simulink model "model_min_mine"  (R2018a)
settings: Solver=ode45  StartTime=0.0  StopTime=20  RelTol=1e-3
(part 9 of 10)

== system model_min_mine/5 систем підйому/6/7-періодні/7-ми періодна пр/Subsystem3 ==
  t1 : Inport
  t : Inport  Port=2
  a1 : Inport  Port=3
  Constant5 : Constant
  Scope2 : Scope
  Sum4 : Sum  Inputs=|+-  SaturateOnIntegerOverflow=on
  Switch1 : Switch  Criteria=u2 ~= 0  RndMeth=Zero  SaturateOnIntegerOverflow=on
  Генераці : Subsystem  TreatAsAtomicUnit=on
  Out1 : Outport
  wires:
  Генераці/1(Out1) -> Switch1/2
  Sum4/1 -> Генераці/Trigger
  Constant5/1 -> Генераці/1(In1)
  t/1 -> Sum4/2
  t1/1 -> Sum4/1
  Switch1/1 -> Out1/1, Scope2/1
  a1/1 -> Switch1/1

== system model_min_mine/5 систем підйому/6/7-періодні/7-ми періодна пр/Subsystem6 ==
  Сума t : Inport
  t : Inport  Port=2
  a : Inport  Port=3
  Constant5 : Constant
  Sum4 : Sum  Inputs=|+-  SaturateOnIntegerOverflow=on
  Switch1 : Switch  Criteria=u2 ~= 0  RndMeth=Zero  SaturateOnIntegerOverflow=on
  Генераці : Subsystem  TreatAsAtomicUnit=on
  Out1 : Outport
  wires:
  Генераці/1(Out1) -> Switch1/2
  Sum4/1 -> Генераці/Trigger
  Constant5/1 -> Генераці/1(In1)
  t/1 -> Sum4/2
  Сума t/1 -> Sum4/1
  Switch1/1 -> Out1/1
  a/1 -> Switch1/3

== system model_min_mine/5 систем підйому/6/7-періодні/7-ми періодна пр/Допоміжний ==
  t1 : Inport
  t : Inport  Port=2
  a1 : Inport  Port=3
  Constant5 : Constant
  Scope2 : Scope
  Sum4 : Sum  Inputs=|+-  SaturateOnIntegerOverflow=on
  Switch1 : Switch  Criteria=u2 ~= 0  RndMeth=Zero  SaturateOnIntegerOverflow=on
  Генераці : Subsystem  TreatAsAtomicUnit=on
  Out1 : Outport
  wires:
  Генераці/1(Out1) -> Switch1/2
  Sum4/1 -> Генераці/Trigger
  Constant5/1 -> Генераці/1(In1)
  t/1 -> Sum4/2
  t1/1 -> Sum4/1
  Switch1/1 -> Out1/1, Scope2/1
  a1/1 -> Switch1/1

== system model_min_mine/5 систем підйому/6/7-періодні/7-ми періодна пр/Допоміжний1 ==
  t1 : Inport
  t : Inport  Port=2
  a1 : Inport  Port=3
  Constant5 : Constant
  Scope2 : Scope
  Sum4 : Sum  Inputs=|+-  SaturateOnIntegerOverflow=on
  Switch1 : Switch  Criteria=u2 ~= 0  RndMeth=Zero  SaturateOnIntegerOverflow=on
  Генераці : Subsystem  TreatAsAtomicUnit=on
  Out1 : Outport
  wires:
  Генераці/1(Out1) -> Switch1/2
  Sum4/1 -> Генераці/Trigger
  Constant5/1 -> Генераці/1(In1)
  t/1 -> Sum4/2
  t1/1 -> Sum4/1
  Switch1/1 -> Out1/1, Scope2/1
  a1/1 -> Switch1/3

== system model_min_mine/5 систем підйому/6/7-періодні/7-ми періодна пр/постійні ==
  Sum1 : Sum  Inputs=|+++++++  SaturateOnIntegerOverflow=on
  Sum2 : Sum  Inputs=|+++  SaturateOnIntegerOverflow=on
  Sum3 : Sum  Inputs=|+++  SaturateOnIntegerOverflow=on
  Sum4 : Sum  Inputs=|++  SaturateOnIntegerOverflow=on
  a1 : Constant  Value=0.5
  a2 : Constant  Value=1.5
  "a4 " : Constant  Value=-1.5
  a5 : Constant  Value=-0.5
  t1 : Constant  Value=0.5
  "t1/ " : Constant  Value=0.5
  t2 : Constant  Value=3.5
  t3 : Constant  Value=8
  t4 : Constant  Value=3.5
  "t4/ " : Constant  Value=0.5
  t5 : Constant  Value=0.5
  Out1 : Outport
  Out2 : Outport  Port=2
  Out3 : Outport  Port=3
  Out4 : Outport  Port=4
  Out5 : Outport  Port=5
  Out6 : Outport  Port=6
  Out7 : Outport  Port=7
  Out8 : Outport  Port=8
  Out9 : Outport  Port=9
  Out10 : Outport  Port=10
  Out11 : Outport  Port=11
  wires:
  a1/1 -> Out1/1
  "a4 "/1 -> Out3/1
  a5/1 -> Out4/1
  a2/1 -> Out2/1
  t1/1 -> Out5/1, Sum1/1, Sum2/1, Sum4/1
  t3/1 -> Sum1/3, Sum2/3
  t2/1 -> Out6/1, Sum1/2, Sum2/2
  t5/1 -> Sum1/5
  t4/1 -> Out7/1, Sum1/4, Sum3/1
  Sum1/1 -> Out9/1
  Sum2/1 -> Out10/1, Sum3/2
  Sum3/1 -> Out8/1
  "t4/ "/1 -> Sum3/3, Sum1/6
  "t1/ "/1 -> Sum1/7, Sum4/2
  Sum4/1 -> Out11/1

== system model_min_mine/5 систем підйому/1/5-періодні/криво/Subsystem/Генераці ==
  In1 : Inport
  Trigger : TriggerPort  TriggerType=either  VariantControl=(inherit)  ShowOutputPort=on
  Out1 : Outport
  wires:
  In1/1 -> Out1/1

== system model_min_mine/5 систем підйому/1/5-періодні/криво/Subsystem1/Генераці ==
  In1 : Inport
  Trigger : TriggerPort  TriggerType=either  VariantControl=(inherit)  ShowOutputPort=on
  Out1 : Outport
  wires:
  In1/1 -> Out1/1

== system model_min_mine/5 систем підйому/1/5-періодні/криво/Subsystem2/Генераці ==
  In1 : Inport
  Trigger : TriggerPort  TriggerType=either  VariantControl=(inherit)  ShowOutputPort=on
  Out1 : Outport
  wires:
  In1/1 -> Out1/1

== system model_min_mine/5 систем підйому/1/5-періодні/криво/Subsystem3/Генераці ==
  In1 : Inport
  Trigger : TriggerPort  TriggerType=either  VariantControl=(inherit)  ShowOutputPort=on
  Out1 : Outport
  wires:
  In1/1 -> Out1/1

== system model_min_mine/5 систем підйому/1/5-періодні/криво/Subsystem6/Генераці ==
  In1 : Inport
  Trigger : TriggerPort  TriggerType=either  VariantControl=(inherit)  ShowOutputPort=on
  Out1 : Outport
  wires:
  In1/1 -> Out1/1

== system model_min_mine/5 систем підйому/1/5-періодні/криво/Допоміжний/Генераці ==
  In1 : Inport
  Trigger : TriggerPort  TriggerType=either  VariantControl=(inherit)  ShowOutputPort=on
  Out1 : Outport
  wires:
  In1/1 -> Out1/1

== system model_min_mine/5 систем підйому/1/5-періодні/криво/Допоміжний1/Генераці ==
  In1 : Inport
  Trigger : TriggerPort  TriggerType=either  VariantControl=(inherit)  ShowOutputPort=on
  Out1 : Outport
  wires:
  In1/1 -> Out1/1

== system model_min_mine/5 систем підйому/1/5-періодні/пр/Subsystem/Генераці ==
  In1 : Inport
  Trigger : TriggerPort  TriggerType=either  VariantControl=(inherit)  ShowOutputPort=on
  Out1 : Outport
  wires:
  In1/1 -> Out1/1

== system model_min_mine/5 систем підйому/1/5-періодні/пр/Subsystem1/Генераці ==
  In1 : Inport
  Trigger : TriggerPort  TriggerType=either  VariantControl=(inherit)  ShowOutputPort=on
  Out1 : Outport
  wires:
  In1/1 -> Out1/1

== system model_min_mine/5 систем підйому/1/5-періодні/пр/Subsystem4/Генераці ==
  In1 : Inport
  Trigger : TriggerPort  TriggerType=either  VariantControl=(inherit)  ShowOutputPort=on
  Out1 : Outport
  wires:
  In1/1 -> Out1/1

== system model_min_mine/5 систем підйому/1/5-періодні/пр/Subsystem5/Генераці ==
  In1 : Inport
  Trigger : TriggerPort  TriggerType=either  VariantControl=(inherit)  ShowOutputPort=on
  Out1 : Outport
  wires:
  In1/1 -> Out1/1

== system model_min_mine/5 систем підйому/1/5-періодні/пр/Subsystem6/Генераці ==
  In1 : Inport
  Trigger : TriggerPort  TriggerType=either  VariantControl=(inherit)  ShowOutputPort=on
  Out1 : Outport
  wires:
  In1/1 -> Out1/1

== system model_min_mine/5 систем підйому/1/5-періодні/пр/Допоміжний/Генераці ==
  In1 : Inport
  Trigger : TriggerPort  TriggerType=either  VariantControl=(inherit)  ShowOutputPort=on
  Out1 : Outport
  wires:
  In1/1 -> Out1/1

== system model_min_mine/5 систем підйому/1/5-періодні/пр/Допоміжний -1/Генераці ==
  In1 : Inport
  Trigger : TriggerPort  TriggerType=either  VariantControl=(inherit)  ShowOutputPort=on
  Out1 : Outport
  wires:
  In1/1 -> Out1/1

== system model_min_mine/5 систем підйому/1/5-періодні/пр/Допоміжний -2/Генераці ==
  In1 : Inport
  Trigger : TriggerPort  TriggerType=either  VariantControl=(inherit)  ShowOutputPort=on
  Out1 : Outport
  wires:
  In1/1 -> Out1/1

== system model_min_mine/5 систем підйому/1/5-періодні/пр/Допоміжний -3/Генераці ==
  In1 : Inport
  Trigger : TriggerPort  TriggerType=either  VariantControl=(inherit)  ShowOutputPort=on
  Out1 : Outport
  wires:
  In1/1 -> Out1/1

== system model_min_mine/5 систем підйому/1/5-періодні/пр/Допоміжний -4/Генераці ==
  In1 : Inport
  Trigger : TriggerPort  TriggerType=either  VariantControl=(inherit)  ShowOutputPort=on
  Out1 : Outport
  wires:
  In1/1 -> Out1/1

== system model_min_mine/5 систем підйому/1/6-періодні/6-ти періодна криволінійна/Subsystem/Генераці ==
  In1 : Inport
  Trigger : TriggerPort  TriggerType=either  VariantControl=(inherit)  ShowOutputPort=on
  Out1 : Outport
  wires:
  In1/1 -> Out1/1

== system model_min_mine/5 систем підйому/1/6-періодні/6-ти періодна криволінійна/Subsystem3/Генераці ==
  In1 : Inport
  Trigger : TriggerPort  TriggerType=either  VariantControl=(inherit)  ShowOutputPort=on
  Out1 : Outport
  wires:
  In1/1 -> Out1/1

== system model_min_mine/5 систем підйому/1/6-періодні/6-ти періодна криволінійна/Subsystem6/Генераці ==
  In1 : Inport
  Trigger : TriggerPort  TriggerType=either  VariantControl=(inherit)  ShowOutputPort=on
  Out1 : Outport
  wires:
  In1/1 -> Out1/1

== system model_min_mine/5 систем підйому/1/6-періодні/6-ти періодна криволінійна/Допоміжний/Генераці ==
  In1 : Inport
  Trigger : TriggerPort  TriggerType=either  VariantControl=(inherit)  ShowOutputPort=on
  Out1 : Outport
  wires:
  In1/1 -> Out1/1

== system model_min_mine/5 систем підйому/1/6-періодні/6-ти періодна криволінійна/Допоміжний1/Генераці ==
  In1 : Inport
  Trigger : TriggerPort  TriggerType=either  VariantControl=(inherit)  ShowOutputPort=on
  Out1 : Outport
  wires:
  In1/1 -> Out1/1

== system model_min_mine/5 систем підйому/1/6-періодні/6-ти періодна пр/Subsystem/Генераці ==
  In1 : Inport
  Trigger : TriggerPort  TriggerType=either  VariantControl=(inherit)  ShowOutputPort=on
  Out1 : Outport
  wires:
  In1/1 -> Out1/1

== system model_min_mine/5 систем підйому/1/6-періодні/6-ти періодна пр/Subsystem1/Генераці ==
  In1 : Inport
  Trigger : TriggerPort  TriggerType=either  VariantControl=(inherit)  ShowOutputPort=on
  Out1 : Outport
  wires:
  In1/1 -> Out1/1

== system model_min_mine/5 систем підйому/1/6-періодні/6-ти періодна пр/Subsystem2/Генераці ==
  In1 : Inport
  Trigger : TriggerPort  TriggerType=either  VariantControl=(inherit)  ShowOutputPort=on
  Out1 : Outport
  wires:
  In1/1 -> Out1/1

== system model_min_mine/5 систем підйому/1/6-періодні/6-ти періодна пр/Subsystem3/Генераці ==
  In1 : Inport
  Trigger : TriggerPort  TriggerType=either  VariantControl=(inherit)  ShowOutputPort=on
  Out1 : Outport
  wires:
  In1/1 -> Out1/1

== system model_min_mine/5 систем підйому/1/6-періодні/6-ти періодна пр/Subsystem6/Генераці ==
  In1 : Inport
  Trigger : TriggerPort  TriggerType=either  VariantControl=(inherit)  ShowOutputPort=on
  Out1 : Outport
  wires:
  In1/1 -> Out1/1

== system model_min_mine/5 систем підйому/1/6-періодні/6-ти періодна пр/Допоміжний/Генераці ==
  In1 : Inport
  Trigger : TriggerPort  TriggerType=either  VariantControl=(inherit)  ShowOutputPort=on
  Out1 : Outport
  wires:
  In1/1 -> Out1/1

== system model_min_mine/5 систем підйому/1/6-періодні/6-ти періодна пр/Допоміжний1/Генераці ==
  In1 : Inport
  Trigger : TriggerPort  TriggerType=either  VariantControl=(inherit)  ShowOutputPort=on
  Out1 : Outport
  wires:
  In1/1 -> Out1/1

== system model_min_mine/5 систем підйому/1/7-періодні/7-ми періодна криволінійна/Subsystem/Генераці ==
  In1 : Inport
  Trigger : TriggerPort  TriggerType=either  VariantControl=(inherit)  ShowOutputPort=on
  Out1 : Outport
  wires:
  In1/1 -> Out1/1

== system model_min_mine/5 систем підйому/1/7-періодні/7-ми періодна криволінійна/Subsystem3/Генераці ==
  In1 : Inport
  Trigger : TriggerPort  TriggerType=either  VariantControl=(inherit)  ShowOutputPort=on
  Out1 : Outport
  wires:
  In1/1 -> Out1/1

== system model_min_mine/5 систем підйому/1/7-періодні/7-ми періодна криволінійна/Subsystem6/Генераці ==
  In1 : Inport
  Trigger : TriggerPort  TriggerType=either  VariantControl=(inherit)  ShowOutputPort=on
  Out1 : Outport
  wires:
  In1/1 -> Out1/1

== system model_min_mine/5 систем підйому/1/7-періодні/7-ми періодна криволінійна/Допоміжний/Генераці ==
  In1 : Inport
  Trigger : TriggerPort  TriggerType=either  VariantControl=(inherit)  ShowOutputPort=on
  Out1 : Outport
  wires:
  In1/1 -> Out1/1

== system model_min_mine/5 систем підйому/1/7-періодні/7-ми періодна криволінійна/Допоміжний1/Генераці ==
  In1 : Inport
  Trigger : TriggerPort  TriggerType=either  VariantControl=(inherit)  ShowOutputPort=on
  Out1 : Outport
  wires:
  In1/1 -> Out1/1

== system model_min_mine/5 систем підйому/1/7-періодні/7-ми періодна пр/Subsystem/Генераці ==
  In1 : Inport
  Trigger : TriggerPort  TriggerType=either  VariantControl=(inherit)  ShowOutputPort=on
  Out1 : Outport
  wires:
  In1/1 -> Out1/1

== system model_min_mine/5 систем підйому/1/7-періодні/7-ми періодна пр/Subsystem1/Генераці ==
  In1 : Inport
  Trigger : TriggerPort  TriggerType=either  VariantControl=(inherit)  ShowOutputPort=on
  Out1 : Outport
  wires:
  In1/1 -> Out1/1

== system model_min_mine/5 систем підйому/1/7-періодні/7-ми періодна пр/Subsystem2/Генераці ==
  In1 : Inport
  Trigger : TriggerPort  TriggerType=either  VariantControl=(inherit)  ShowOutputPort=on
  Out1 : Outport
  wires:
  In1/1 -> Out1/1

== system model_min_mine/5 систем підйому/1/7-періодні/7-ми періодна пр/Subsystem3/Генераці ==
  In1 : Inport
  Trigger : TriggerPort  TriggerType=either  VariantControl=(inherit)  ShowOutputPort=on
  Out1 : Outport
  wires:
  In1/1 -> Out1/1

== system model_min_mine/5 систем підйому/1/7-періодні/7-ми періодна пр/Subsystem6/Генераці ==
  In1 : Inport
  Trigger : TriggerPort  TriggerType=either  VariantControl=(inherit)  ShowOutputPort=on
  Out1 : Outport
  wires:
  In1/1 -> Out1/1

== system model_min_mine/5 систем підйому/1/7-періодні/7-ми періодна пр/Допоміжний/Генераці ==
  In1 : Inport
  Trigger : TriggerPort  TriggerType=either  VariantControl=(inherit)  ShowOutputPort=on
  Out1 : Outport
  wires:
  In1/1 -> Out1/1

== system model_min_mine/5 систем підйому/1/7-періодні/7-ми періодна пр/Допоміжний1/Генераці ==
  In1 : Inport
  Trigger : TriggerPort  TriggerType=either  VariantControl=(inherit)  ShowOutputPort=on
  Out1 : Outport
  wires:
  In1/1 -> Out1/1

== system model_min_mine/5 систем підйому/2/5-періодні/криво/Subsystem/Генераці ==
  In1 : Inport
  Trigger : TriggerPort  TriggerType=either  VariantControl=(inherit)  ShowOutputPort=on
  Out1 : Outport
  wires:
  In1/1 -> Out1/1

== system model_min_mine/5 систем підйому/2/5-періодні/криво/Subsystem1/Генераці ==
  In1 : Inport
  Trigger : TriggerPort  TriggerType=either  VariantControl=(inherit)  ShowOutputPort=on
  Out1 : Outport
  wires:
  In1/1 -> Out1/1

== system model_min_mine/5 систем підйому/2/5-періодні/криво/Subsystem2/Генераці ==
  In1 : Inport
  Trigger : TriggerPort  TriggerType=either  VariantControl=(inherit)  ShowOutputPort=on
  Out1 : Outport
  wires:
  In1/1 -> Out1/1

== system model_min_mine/5 систем підйому/2/5-періодні/криво/Subsystem3/Генераці ==
  In1 : Inport
  Trigger : TriggerPort  TriggerType=either  VariantControl=(inherit)  ShowOutputPort=on
  Out1 : Outport
  wires:
  In1/1 -> Out1/1

== system model_min_mine/5 систем підйому/2/5-періодні/криво/Subsystem6/Генераці ==
  In1 : Inport
  Trigger : TriggerPort  TriggerType=either  VariantControl=(inherit)  ShowOutputPort=on
  Out1 : Outport
  wires:
  In1/1 -> Out1/1

== system model_min_mine/5 систем підйому/2/5-періодні/криво/Допоміжний/Генераці ==
  In1 : Inport
  Trigger : TriggerPort  TriggerType=either  VariantControl=(inherit)  ShowOutputPort=on
  Out1 : Outport
  wires:
  In1/1 -> Out1/1

== system model_min_mine/5 систем підйому/2/5-періодні/криво/Допоміжний1/Генераці ==
  In1 : Inport
  Trigger : TriggerPort  TriggerType=either  VariantControl=(inherit)  ShowOutputPort=on
  Out1 : Outport
  wires:
  In1/1 -> Out1/1

== system model_min_mine/5 систем підйому/2/5-періодні/пр/Subsystem/Генераці ==
  In1 : Inport
  Trigger : TriggerPort  TriggerType=either  VariantControl=(inherit)  ShowOutputPort=on
  Out1 : Outport
  wires:
  In1/1 -> Out1/1

== system model_min_mine/5 систем підйому/2/5-періодні/пр/Subsystem1/Генераці ==
  In1 : Inport
  Trigger : TriggerPort  TriggerType=either  VariantControl=(inherit)  ShowOutputPort=on
  Out1 : Outport
  wires:
  In1/1 -> Out1/1

== system model_min_mine/5 систем підйому/2/5-періодні/пр/Subsystem4/Генераці ==
  In1 : Inport
  Trigger : TriggerPort  TriggerType=either  VariantControl=(inherit)  ShowOutputPort=on
  Out1 : Outport
  wires:
  In1/1 -> Out1/1

== system model_min_mine/5 систем підйому/2/5-періодні/пр/Subsystem5/Генераці ==
  In1 : Inport
  Trigger : TriggerPort  TriggerType=either  VariantControl=(inherit)  ShowOutputPort=on
  Out1 : Outport
  wires:
  In1/1 -> Out1/1

== system model_min_mine/5 систем підйому/2/5-періодні/пр/Subsystem6/Генераці ==
  In1 : Inport
  Trigger : TriggerPort  TriggerType=either  VariantControl=(inherit)  ShowOutputPort=on
  Out1 : Outport
  wires:
  In1/1 -> Out1/1

== system model_min_mine/5 систем підйому/2/5-періодні/пр/Допоміжний/Генераці ==
  In1 : Inport
  Trigger : TriggerPort  TriggerType=either  VariantControl=(inherit)  ShowOutputPort=on
  Out1 : Outport
  wires:
  In1/1 -> Out1/1

== system model_min_mine/5 систем підйому/2/5-періодні/пр/Допоміжний -1/Генераці ==
  In1 : Inport
  Trigger : TriggerPort  TriggerType=either  VariantControl=(inherit)  ShowOutputPort=on
  Out1 : Outport
  wires:
  In1/1 -> Out1/1

== system model_min_mine/5 систем підйому/2/5-періодні/пр/Допоміжний -2/Генераці ==
  In1 : Inport
  Trigger : TriggerPort  TriggerType=either  VariantControl=(inherit)  ShowOutputPort=on
  Out1 : Outport
  wires:
  In1/1 -> Out1/1

== system model_min_mine/5 систем підйому/2/5-періодні/пр/Допоміжний -3/Генераці ==
  In1 : Inport
  Trigger : TriggerPort  TriggerType=either  VariantControl=(inherit)  ShowOutputPort=on
  Out1 : Outport
  wires:
  In1/1 -> Out1/1

== system model_min_mine/5 систем підйому/2/5-періодні/пр/Допоміжний -4/Генераці ==
  In1 : Inport
  Trigger : TriggerPort  TriggerType=either  VariantControl=(inherit)  ShowOutputPort=on
  Out1 : Outport
  wires:
  In1/1 -> Out1/1

== system model_min_mine/5 систем підйому/2/6-періодні/6-ти періодна криволінійна/Subsystem/Генераці ==
  In1 : Inport
  Trigger : TriggerPort  TriggerType=either  VariantControl=(inherit)  ShowOutputPort=on
  Out1 : Outport
  wires:
  In1/1 -> Out1/1

== system model_min_mine/5 систем підйому/2/6-періодні/6-ти періодна криволінійна/Subsystem3/Генераці ==
  In1 : Inport
  Trigger : TriggerPort  TriggerType=either  VariantControl=(inherit)  ShowOutputPort=on
  Out1 : Outport
  wires:
  In1/1 -> Out1/1

== system model_min_mine/5 систем підйому/2/6-періодні/6-ти періодна криволінійна/Subsystem6/Генераці ==
  In1 : Inport
  Trigger : TriggerPort  TriggerType=either  VariantControl=(inherit)  ShowOutputPort=on
  Out1 : Outport
  wires:
  In1/1 -> Out1/1

== system model_min_mine/5 систем підйому/2/6-періодні/6-ти періодна криволінійна/Допоміжний/Генераці ==
  In1 : Inport
  Trigger : TriggerPort  TriggerType=either  VariantControl=(inherit)  ShowOutputPort=on
  Out1 : Outport
  wires:
  In1/1 -> Out1/1

== system model_min_mine/5 систем підйому/2/6-періодні/6-ти періодна криволінійна/Допоміжний1/Генераці ==
  In1 : Inport
  Trigger : TriggerPort  TriggerType=either  VariantControl=(inherit)  ShowOutputPort=on
  Out1 : Outport
  wires:
  In1/1 -> Out1/1

== system model_min_mine/5 систем підйому/2/6-періодні/6-ти періодна пр/Subsystem/Генераці ==
  In1 : Inport
  Trigger : TriggerPort  TriggerType=either  VariantControl=(inherit)  ShowOutputPort=on
  Out1 : Outport
  wires:
  In1/1 -> Out1/1

== system model_min_mine/5 систем підйому/2/6-періодні/6-ти періодна пр/Subsystem1/Генераці ==
  In1 : Inport
  Trigger : TriggerPort  TriggerType=either  VariantControl=(inherit)  ShowOutputPort=on
  Out1 : Outport
  wires:
  In1/1 -> Out1/1

== system model_min_mine/5 систем підйому/2/6-періодні/6-ти періодна пр/Subsystem2/Генераці ==
  In1 : Inport
  Trigger : TriggerPort  TriggerType=either  VariantControl=(inherit)  ShowOutputPort=on
  Out1 : Outport
  wires:
  In1/1 -> Out1/1

== system model_min_mine/5 систем підйому/2/6-періодні/6-ти періодна пр/Subsystem3/Генераці ==
  In1 : Inport
  Trigger : TriggerPort  TriggerType=either  VariantControl=(inherit)  ShowOutputPort=on
  Out1 : Outport
  wires:
  In1/1 -> Out1/1

== system model_min_mine/5 систем підйому/2/6-періодні/6-ти періодна пр/Subsystem6/Генераці ==
  In1 : Inport
  Trigger : TriggerPort  TriggerType=either  VariantControl=(inherit)  ShowOutputPort=on
  Out1 : Outport
  wires:
  In1/1 -> Out1/1

== system model_min_mine/5 систем підйому/2/6-періодні/6-ти періодна пр/Допоміжний/Генераці ==
  In1 : Inport
  Trigger : TriggerPort  TriggerType=either  VariantControl=(inherit)  ShowOutputPort=on
  Out1 : Outport
  wires:
  In1/1 -> Out1/1

== system model_min_mine/5 систем підйому/2/6-періодні/6-ти періодна пр/Допоміжний1/Генераці ==
  In1 : Inport
  Trigger : TriggerPort  TriggerType=either  VariantControl=(inherit)  ShowOutputPort=on
  Out1 : Outport
  wires:
  In1/1 -> Out1/1

== system model_min_mine/5 систем підйому/2/7-періодні/7-ми періодна криволінійна/Subsystem/Генераці ==
  In1 : Inport
  Trigger : TriggerPort  TriggerType=either  VariantControl=(inherit)  ShowOutputPort=on
  Out1 : Outport
  wires:
  In1/1 -> Out1/1

== system model_min_mine/5 систем підйому/2/7-періодні/7-ми періодна криволінійна/Subsystem3/Генераці ==
  In1 : Inport
  Trigger : TriggerPort  TriggerType=either  VariantControl=(inherit)  ShowOutputPort=on
  Out1 : Outport
  wires:
  In1/1 -> Out1/1

== system model_min_mine/5 систем підйому/2/7-періодні/7-ми періодна криволінійна/Subsystem6/Генераці ==
  In1 : Inport
  Trigger : TriggerPort  TriggerType=either  VariantControl=(inherit)  ShowOutputPort=on
  Out1 : Outport
  wires:
  In1/1 -> Out1/1

== system model_min_mine/5 систем підйому/2/7-періодні/7-ми періодна криволінійна/Допоміжний/Генераці ==
  In1 : Inport
  Trigger : TriggerPort  TriggerType=either  VariantControl=(inherit)  ShowOutputPort=on
  Out1 : Outport
  wires:
  In1/1 -> Out1/1

== system model_min_mine/5 систем підйому/2/7-періодні/7-ми періодна криволінійна/Допоміжний1/Генераці ==
  In1 : Inport
  Trigger : TriggerPort  TriggerType=either  VariantControl=(inherit)  ShowOutputPort=on
  Out1 : Outport
  wires:
  In1/1 -> Out1/1

== system model_min_mine/5 систем підйому/2/7-періодні/7-ми періодна пр/Subsystem/Генераці ==
  In1 : Inport
  Trigger : TriggerPort  TriggerType=either  VariantControl=(inherit)  ShowOutputPort=on
  Out1 : Outport
  wires:
  In1/1 -> Out1/1

== system model_min_mine/5 систем підйому/2/7-періодні/7-ми періодна пр/Subsystem1/Генераці ==
  In1 : Inport
  Trigger : TriggerPort  TriggerType=either  VariantControl=(inherit)  ShowOutputPort=on
  Out1 : Outport
  wires:
  In1/1 -> Out1/1

== system model_min_mine/5 систем підйому/2/7-періодні/7-ми періодна пр/Subsystem2/Генераці ==
  In1 : Inport
  Trigger : TriggerPort  TriggerType=either  VariantControl=(inherit)  ShowOutputPort=on
  Out1 : Outport
  wires:
  In1/1 -> Out1/1

== system model_min_mine/5 систем підйому/2/7-періодні/7-ми періодна пр/Subsystem3/Генераці ==
  In1 : Inport
  Trigger : TriggerPort  TriggerType=either  VariantControl=(inherit)  ShowOutputPort=on
  Out1 : Outport
  wires:
  In1/1 -> Out1/1

== system model_min_mine/5 систем підйому/2/7-періодні/7-ми періодна пр/Subsystem6/Генераці ==
  In1 : Inport
  Trigger : TriggerPort  TriggerType=either  VariantControl=(inherit)  ShowOutputPort=on
  Out1 : Outport
  wires:
  In1/1 -> Out1/1

== system model_min_mine/5 систем підйому/2/7-періодні/7-ми періодна пр/Допоміжний/Генераці ==
  In1 : Inport
  Trigger : TriggerPort  TriggerType=either  VariantControl=(inherit)  ShowOutputPort=on
  Out1 : Outport
  wires:
  In1/1 -> Out1/1

== system model_min_mine/5 систем підйому/2/7-періодні/7-ми періодна пр/Допоміжний1/Генераці ==
  In1 : Inport
  Trigger : TriggerPort  TriggerType=either  VariantControl=(inherit)  ShowOutputPort=on
  Out1 : Outport
  wires:
  In1/1 -> Out1/1

== system model_min_mine/5 систем підйому/3/5-періодні/криво/Subsystem/Генераці ==
  In1 : Inport
  Trigger : TriggerPort  TriggerType=either  VariantControl=(inherit)  ShowOutputPort=on
  Out1 : Outport
  wires:
  In1/1 -> Out1/1

== system model_min_mine/5 систем підйому/3/5-періодні/криво/Subsystem1/Генераці ==
  In1 : Inport
  Trigger : TriggerPort  TriggerType=either  VariantControl=(inherit)  ShowOutputPort=on
  Out1 : Outport
  wires:
  In1/1 -> Out1/1

== system model_min_mine/5 систем підйому/3/5-періодні/криво/Subsystem2/Генераці ==
  In1 : Inport
  Trigger : TriggerPort  TriggerType=either  VariantControl=(inherit)  ShowOutputPort=on
  Out1 : Outport
  wires:
  In1/1 -> Out1/1

== system model_min_mine/5 систем підйому/3/5-періодні/криво/Subsystem3/Генераці ==
  In1 : Inport
  Trigger : TriggerPort  TriggerType=either  VariantControl=(inherit)  ShowOutputPort=on
  Out1 : Outport
  wires:
  In1/1 -> Out1/1

== system model_min_mine/5 систем підйому/3/5-періодні/криво/Subsystem6/Генераці ==
  In1 : Inport
  Trigger : TriggerPort  TriggerType=either  VariantControl=(inherit)  ShowOutputPort=on
  Out1 : Outport
  wires:
  In1/1 -> Out1/1

== system model_min_mine/5 систем підйому/3/5-періодні/криво/Допоміжний/Генераці ==
  In1 : Inport
  Trigger : TriggerPort  TriggerType=either  VariantControl=(inherit)  ShowOutputPort=on
  Out1 : Outport
  wires:
  In1/1 -> Out1/1

== system model_min_mine/5 систем підйому/3/5-періодні/криво/Допоміжний1/Генераці ==
  In1 : Inport
  Trigger : TriggerPort  TriggerType=either  VariantControl=(inherit)  ShowOutputPort=on
  Out1 : Outport
  wires:
  In1/1 -> Out1/1

== system model_min_mine/5 систем підйому/3/5-періодні/пр/Subsystem/Генераці ==
  In1 : Inport
  Trigger : TriggerPort  TriggerType=either  VariantControl=(inherit)  ShowOutputPort=on
  Out1 : Outport
  wires:
  In1/1 -> Out1/1

== system model_min_mine/5 систем підйому/3/5-періодні/пр/Subsystem1/Генераці ==
  In1 : Inport
  Trigger : TriggerPort  TriggerType=either  VariantControl=(inherit)  ShowOutputPort=on
  Out1 : Outport
  wires:
  In1/1 -> Out1/1

== system model_min_mine/5 систем підйому/3/5-періодні/пр/Subsystem4/Генераці ==
  In1 : Inport
  Trigger : TriggerPort  TriggerType=either  VariantControl=(inherit)  ShowOutputPort=on
  Out1 : Outport
  wires:
  In1/1 -> Out1/1

== system model_min_mine/5 систем підйому/3/5-періодні/пр/Subsystem5/Генераці ==
  In1 : Inport
  Trigger : TriggerPort  TriggerType=either  VariantControl=(inherit)  ShowOutputPort=on
  Out1 : Outport
  wires:
  In1/1 -> Out1/1

== system model_min_mine/5 систем підйому/3/5-періодні/пр/Subsystem6/Генераці ==
  In1 : Inport
  Trigger : TriggerPort  TriggerType=either  VariantControl=(inherit)  ShowOutputPort=on
  Out1 : Outport
  wires:
  In1/1 -> Out1/1

== system model_min_mine/5 систем підйому/3/5-періодні/пр/Допоміжний/Генераці ==
  In1 : Inport
  Trigger : TriggerPort  TriggerType=either  VariantControl=(inherit)  ShowOutputPort=on
  Out1 : Outport
  wires:
  In1/1 -> Out1/1

== system model_min_mine/5 систем підйому/3/5-періодні/пр/Допоміжний -1/Генераці ==
  In1 : Inport
  Trigger : TriggerPort  TriggerType=either  VariantControl=(inherit)  ShowOutputPort=on
  Out1 : Outport
  wires:
  In1/1 -> Out1/1

== system model_min_mine/5 систем підйому/3/5-періодні/пр/Допоміжний -2/Генераці ==
  In1 : Inport
  Trigger : TriggerPort  TriggerType=either  VariantControl=(inherit)  ShowOutputPort=on
  Out1 : Outport
  wires:
  In1/1 -> Out1/1

== system model_min_mine/5 систем підйому/3/5-періодні/пр/Допоміжний -3/Генераці ==
  In1 : Inport
  Trigger : TriggerPort  TriggerType=either  VariantControl=(inherit)  ShowOutputPort=on
  Out1 : Outport
  wires:
  In1/1 -> Out1/1

== system model_min_mine/5 систем підйому/3/5-періодні/пр/Допоміжний -4/Генераці ==
  In1 : Inport
  Trigger : TriggerPort  TriggerType=either  VariantControl=(inherit)  ShowOutputPort=on
  Out1 : Outport
  wires:
  In1/1 -> Out1/1

== system model_min_mine/5 систем підйому/3/6-періодні/6-ти періодна криволінійна/Subsystem/Генераці ==
  In1 : Inport
  Trigger : TriggerPort  TriggerType=either  VariantControl=(inherit)  ShowOutputPort=on
  Out1 : Outport
  wires:
  In1/1 -> Out1/1

== system model_min_mine/5 систем підйому/3/6-періодні/6-ти періодна криволінійна/Subsystem3/Генераці ==
  In1 : Inport
  Trigger : TriggerPort  TriggerType=either  VariantControl=(inherit)  ShowOutputPort=on
  Out1 : Outport
  wires:
  In1/1 -> Out1/1

== system model_min_mine/5 систем підйому/3/6-періодні/6-ти періодна криволінійна/Subsystem6/Генераці ==
  In1 : Inport
  Trigger : TriggerPort  TriggerType=either  VariantControl=(inherit)  ShowOutputPort=on
  Out1 : Outport
  wires:
  In1/1 -> Out1/1

== system model_min_mine/5 систем підйому/3/6-періодні/6-ти періодна криволінійна/Допоміжний/Генераці ==
  In1 : Inport
  Trigger : TriggerPort  TriggerType=either  VariantControl=(inherit)  ShowOutputPort=on
  Out1 : Outport
  wires:
  In1/1 -> Out1/1

== system model_min_mine/5 систем підйому/3/6-періодні/6-ти періодна криволінійна/Допоміжний1/Генераці ==
  In1 : Inport
  Trigger : TriggerPort  TriggerType=either  VariantControl=(inherit)  ShowOutputPort=on
  Out1 : Outport
  wires:
  In1/1 -> Out1/1

== system model_min_mine/5 систем підйому/3/6-періодні/6-ти періодна пр/Subsystem/Генераці ==
  In1 : Inport
  Trigger : TriggerPort  TriggerType=either  VariantControl=(inherit)  ShowOutputPort=on
  Out1 : Outport
  wires:
  In1/1 -> Out1/1

== system model_min_mine/5 систем підйому/3/6-періодні/6-ти періодна пр/Subsystem1/Генераці ==
  In1 : Inport
  Trigger : TriggerPort  TriggerType=either  VariantControl=(inherit)  ShowOutputPort=on
  Out1 : Outport
  wires:
  In1/1 -> Out1/1

== system model_min_mine/5 систем підйому/3/6-періодні/6-ти періодна пр/Subsystem2/Генераці ==
  In1 : Inport
  Trigger : TriggerPort  TriggerType=either  VariantControl=(inherit)  ShowOutputPort=on
  Out1 : Outport
  wires:
  In1/1 -> Out1/1

== system model_min_mine/5 систем підйому/3/6-періодні/6-ти періодна пр/Subsystem3/Генераці ==
  In1 : Inport
  Trigger : TriggerPort  TriggerType=either  VariantControl=(inherit)  ShowOutputPort=on
  Out1 : Outport
  wires:
  In1/1 -> Out1/1

== system model_min_mine/5 систем підйому/3/6-періодні/6-ти періодна пр/Subsystem6/Генераці ==
  In1 : Inport
  Trigger : TriggerPort  TriggerType=either  VariantControl=(inherit)  ShowOutputPort=on
  Out1 : Outport
  wires:
  In1/1 -> Out1/1

== system model_min_mine/5 систем підйому/3/6-періодні/6-ти періодна пр/Допоміжний/Генераці ==
  In1 : Inport
  Trigger : TriggerPort  TriggerType=either  VariantControl=(inherit)  ShowOutputPort=on
  Out1 : Outport
  wires:
  In1/1 -> Out1/1

== system model_min_mine/5 систем підйому/3/6-періодні/6-ти періодна пр/Допоміжний1/Генераці ==
  In1 : Inport
  Trigger : TriggerPort  TriggerType=either  VariantControl=(inherit)  ShowOutputPort=on
  Out1 : Outport
  wires:
  In1/1 -> Out1/1

== system model_min_mine/5 систем підйому/3/7-періодні/7-ми періодна криволінійна/Subsystem/Генераці ==
  In1 : Inport
  Trigger : TriggerPort  TriggerType=either  VariantControl=(inherit)  ShowOutputPort=on
  Out1 : Outport
  wires:
  In1/1 -> Out1/1

== system model_min_mine/5 систем підйому/3/7-періодні/7-ми періодна криволінійна/Subsystem3/Генераці ==
  In1 : Inport
  Trigger : TriggerPort  TriggerType=either  VariantControl=(inherit)  ShowOutputPort=on
  Out1 : Outport
  wires:
  In1/1 -> Out1/1

== system model_min_mine/5 систем підйому/3/7-періодні/7-ми періодна криволінійна/Subsystem6/Генераці ==
  In1 : Inport
  Trigger : TriggerPort  TriggerType=either  VariantControl=(inherit)  ShowOutputPort=on
  Out1 : Outport
  wires:
  In1/1 -> Out1/1

== system model_min_mine/5 систем підйому/3/7-періодні/7-ми періодна криволінійна/Допоміжний/Генераці ==
  In1 : Inport
  Trigger : TriggerPort  TriggerType=either  VariantControl=(inherit)  ShowOutputPort=on
  Out1 : Outport
  wires:
  In1/1 -> Out1/1

== system model_min_mine/5 систем підйому/3/7-періодні/7-ми періодна криволінійна/Допоміжний1/Генераці ==
  In1 : Inport
  Trigger : TriggerPort  TriggerType=either  VariantControl=(inherit)  ShowOutputPort=on
  Out1 : Outport
  wires:
  In1/1 -> Out1/1

== system model_min_mine/5 систем підйому/3/7-періодні/7-ми періодна пр/Subsystem/Генераці ==
  In1 : Inport
  Trigger : TriggerPort  TriggerType=either  VariantControl=(inherit)  ShowOutputPort=on
  Out1 : Outport
  wires:
  In1/1 -> Out1/1

== system model_min_mine/5 систем підйому/3/7-періодні/7-ми періодна пр/Subsystem1/Генераці ==
  In1 : Inport
  Trigger : TriggerPort  TriggerType=either  VariantControl=(inherit)  ShowOutputPort=on
  Out1 : Outport
  wires:
  In1/1 -> Out1/1

== system model_min_mine/5 систем підйому/3/7-періодні/7-ми періодна пр/Subsystem2/Генераці ==
  In1 : Inport
  Trigger : TriggerPort  TriggerType=either  VariantControl=(inherit)  ShowOutputPort=on
  Out1 : Outport
  wires:
  In1/1 -> Out1/1

== system model_min_mine/5 систем підйому/3/7-періодні/7-ми періодна пр/Subsystem3/Генераці ==
  In1 : Inport
  Trigger : TriggerPort  TriggerType=either  VariantControl=(inherit)  ShowOutputPort=on
  Out1 : Outport
  wires:
  In1/1 -> Out1/1

== system model_min_mine/5 систем підйому/3/7-періодні/7-ми періодна пр/Subsystem6/Генераці ==
  In1 : Inport
  Trigger : TriggerPort  TriggerType=either  VariantControl=(inherit)  ShowOutputPort=on
  Out1 : Outport
  wires:
  In1/1 -> Out1/1

== system model_min_mine/5 систем підйому/3/7-періодні/7-ми періодна пр/Допоміжний/Генераці ==
  In1 : Inport
  Trigger : TriggerPort  TriggerType=either  VariantControl=(inherit)  ShowOutputPort=on
  Out1 : Outport
  wires:
  In1/1 -> Out1/1

== system model_min_mine/5 систем підйому/3/7-періодні/7-ми періодна пр/Допоміжний1/Генераці ==
  In1 : Inport
  Trigger : TriggerPort  TriggerType=either  VariantControl=(inherit)  ShowOutputPort=on
  Out1 : Outport
  wires:
  In1/1 -> Out1/1

== system model_min_mine/5 систем підйому/4/5-періодні/криво/Subsystem/Генераці ==
  In1 : Inport
  Trigger : TriggerPort  TriggerType=either  VariantControl=(inherit)  ShowOutputPort=on
  Out1 : Outport
  wires:
  In1/1 -> Out1/1

== system model_min_mine/5 систем підйому/4/5-періодні/криво/Subsystem1/Генераці ==
  In1 : Inport
  Trigger : TriggerPort  TriggerType=either  VariantControl=(inherit)  ShowOutputPort=on
  Out1 : Outport
  wires:
  In1/1 -> Out1/1

== system model_min_mine/5 систем підйому/4/5-періодні/криво/Subsystem2/Генераці ==
  In1 : Inport
  Trigger : TriggerPort  TriggerType=either  VariantControl=(inherit)  ShowOutputPort=on
  Out1 : Outport
  wires:
  In1/1 -> Out1/1

== system model_min_mine/5 систем підйому/4/5-періодні/криво/Subsystem3/Генераці ==
  In1 : Inport
  Trigger : TriggerPort  TriggerType=either  VariantControl=(inherit)  ShowOutputPort=on
  Out1 : Outport
  wires:
  In1/1 -> Out1/1

== system model_min_mine/5 систем підйому/4/5-періодні/криво/Subsystem6/Генераці ==
  In1 : Inport
  Trigger : TriggerPort  TriggerType=either  VariantControl=(inherit)  ShowOutputPort=on
  Out1 : Outport
  wires:
  In1/1 -> Out1/1

== system model_min_mine/5 систем підйому/4/5-періодні/криво/Допоміжний/Генераці ==
  In1 : Inport
  Trigger : TriggerPort  TriggerType=either  VariantControl=(inherit)  ShowOutputPort=on
  Out1 : Outport
  wires:
  In1/1 -> Out1/1

== system model_min_mine/5 систем підйому/4/5-періодні/криво/Допоміжний1/Генераці ==
  In1 : Inport
  Trigger : TriggerPort  TriggerType=either  VariantControl=(inherit)  ShowOutputPort=on
  Out1 : Outport
  wires:
  In1/1 -> Out1/1

== system model_min_mine/5 систем підйому/4/5-періодні/пр/Subsystem/Генераці ==
  In1 : Inport
  Trigger : TriggerPort  TriggerType=either  VariantControl=(inherit)  ShowOutputPort=on
  Out1 : Outport
  wires:
  In1/1 -> Out1/1

== system model_min_mine/5 систем підйому/4/5-періодні/пр/Subsystem1/Генераці ==
  In1 : Inport
  Trigger : TriggerPort  TriggerType=either  VariantControl=(inherit)  ShowOutputPort=on
  Out1 : Outport
  wires:
  In1/1 -> Out1/1

== system model_min_mine/5 систем підйому/4/5-періодні/пр/Subsystem4/Генераці ==
  In1 : Inport
  Trigger : TriggerPort  TriggerType=either  VariantControl=(inherit)  ShowOutputPort=on
  Out1 : Outport
  wires:
  In1/1 -> Out1/1

== system model_min_mine/5 систем підйому/4/5-періодні/пр/Subsystem5/Генераці ==
  In1 : Inport
  Trigger : TriggerPort  TriggerType=either  VariantControl=(inherit)  ShowOutputPort=on
  Out1 : Outport
  wires:
  In1/1 -> Out1/1

== system model_min_mine/5 систем підйому/4/5-періодні/пр/Subsystem6/Генераці ==
  In1 : Inport
  Trigger : TriggerPort  TriggerType=either  VariantControl=(inherit)  ShowOutputPort=on
  Out1 : Outport
  wires:
  In1/1 -> Out1/1

== system model_min_mine/5 систем підйому/4/5-періодні/пр/Допоміжний/Генераці ==
  In1 : Inport
  Trigger : TriggerPort  TriggerType=either  VariantControl=(inherit)  ShowOutputPort=on
  Out1 : Outport
  wires:
  In1/1 -> Out1/1

== system model_min_mine/5 систем підйому/4/5-періодні/пр/Допоміжний -1/Генераці ==
  In1 : Inport
  Trigger : TriggerPort  TriggerType=either  VariantControl=(inherit)  ShowOutputPort=on
  Out1 : Outport
  wires:
  In1/1 -> Out1/1

== system model_min_mine/5 систем підйому/4/5-періодні/пр/Допоміжний -2/Генераці ==
  In1 : Inport
  Trigger : TriggerPort  TriggerType=either  VariantControl=(inherit)  ShowOutputPort=on
  Out1 : Outport
  wires:
  In1/1 -> Out1/1

== system model_min_mine/5 систем підйому/4/5-періодні/пр/Допоміжний -3/Генераці ==
  In1 : Inport
  Trigger : TriggerPort  TriggerType=either  VariantControl=(inherit)  ShowOutputPort=on
  Out1 : Outport
  wires:
  In1/1 -> Out1/1

== system model_min_mine/5 систем підйому/4/5-періодні/пр/Допоміжний -4/Генераці ==
  In1 : Inport
  Trigger : TriggerPort  TriggerType=either  VariantControl=(inherit)  ShowOutputPort=on
  Out1 : Outport
  wires:
  In1/1 -> Out1/1

== system model_min_mine/5 систем підйому/4/6-періодні/6-ти періодна криволінійна/Subsystem/Генераці ==
  In1 : Inport
  Trigger : TriggerPort  TriggerType=either  VariantControl=(inherit)  ShowOutputPort=on
  Out1 : Outport
  wires:
  In1/1 -> Out1/1

== system model_min_mine/5 систем підйому/4/6-періодні/6-ти періодна криволінійна/Subsystem3/Генераці ==
  In1 : Inport
  Trigger : TriggerPort  TriggerType=either  VariantControl=(inherit)  ShowOutputPort=on
  Out1 : Outport
  wires:
  In1/1 -> Out1/1

== system model_min_mine/5 систем підйому/4/6-періодні/6-ти періодна криволінійна/Subsystem6/Генераці ==
  In1 : Inport
  Trigger : TriggerPort  TriggerType=either  VariantControl=(inherit)  ShowOutputPort=on
  Out1 : Outport
  wires:
  In1/1 -> Out1/1

== system model_min_mine/5 систем підйому/4/6-періодні/6-ти періодна криволінійна/Допоміжний/Генераці ==
  In1 : Inport
  Trigger : TriggerPort  TriggerType=either  VariantControl=(inherit)  ShowOutputPort=on
  Out1 : Outport
  wires:
  In1/1 -> Out1/1

== system model_min_mine/5 систем підйому/4/6-періодні/6-ти періодна криволінійна/Допоміжний1/Генераці ==
  In1 : Inport
  Trigger : TriggerPort  TriggerType=either  VariantControl=(inherit)  ShowOutputPort=on
  Out1 : Outport
  wires:
  In1/1 -> Out1/1

== system model_min_mine/5 систем підйому/4/6-періодні/6-ти періодна пр/Subsystem/Генераці ==
  In1 : Inport
  Trigger : TriggerPort  TriggerType=either  VariantControl=(inherit)  ShowOutputPort=on
  Out1 : Outport
  wires:
  In1/1 -> Out1/1

== system model_min_mine/5 систем підйому/4/6-періодні/6-ти періодна пр/Subsystem1/Генераці ==
  In1 : Inport
  Trigger : TriggerPort  TriggerType=either  VariantControl=(inherit)  ShowOutputPort=on
  Out1 : Outport
  wires:
  In1/1 -> Out1/1

== system model_min_mine/5 систем підйому/4/6-періодні/6-ти періодна пр/Subsystem2/Генераці ==
  In1 : Inport
  Trigger : TriggerPort  TriggerType=either  VariantControl=(inherit)  ShowOutputPort=on
  Out1 : Outport
  wires:
  In1/1 -> Out1/1

== system model_min_mine/5 систем підйому/4/6-періодні/6-ти періодна пр/Subsystem3/Генераці ==
  In1 : Inport
  Trigger : TriggerPort  TriggerType=either  VariantControl=(inherit)  ShowOutputPort=on
  Out1 : Outport
  wires:
  In1/1 -> Out1/1

== system model_min_mine/5 систем підйому/4/6-періодні/6-ти періодна пр/Subsystem6/Генераці ==
  In1 : Inport
  Trigger : TriggerPort  TriggerType=either  VariantControl=(inherit)  ShowOutputPort=on
  Out1 : Outport
  wires:
  In1/1 -> Out1/1

== system model_min_mine/5 систем підйому/4/6-періодні/6-ти періодна пр/Допоміжний/Генераці ==
  In1 : Inport
  Trigger : TriggerPort  TriggerType=either  VariantControl=(inherit)  ShowOutputPort=on
  Out1 : Outport
  wires:
  In1/1 -> Out1/1

== system model_min_mine/5 систем підйому/4/6-періодні/6-ти періодна пр/Допоміжний1/Генераці ==
  In1 : Inport
  Trigger : TriggerPort  TriggerType=either  VariantControl=(inherit)  ShowOutputPort=on
  Out1 : Outport
  wires:
  In1/1 -> Out1/1

== system model_min_mine/5 систем підйому/4/7-періодні/7-ми періодна криволінійна/Subsystem/Генераці ==
  In1 : Inport
  Trigger : TriggerPort  TriggerType=either  VariantControl=(inherit)  ShowOutputPort=on
  Out1 : Outport
  wires:
  In1/1 -> Out1/1

== system model_min_mine/5 систем підйому/4/7-періодні/7-ми періодна криволінійна/Subsystem3/Генераці ==
  In1 : Inport
  Trigger : TriggerPort  TriggerType=either  VariantControl=(inherit)  ShowOutputPort=on
  Out1 : Outport
  wires:
  In1/1 -> Out1/1

== system model_min_mine/5 систем підйому/4/7-періодні/7-ми періодна криволінійна/Subsystem6/Генераці ==
  In1 : Inport
  Trigger : TriggerPort  TriggerType=either  VariantControl=(inherit)  ShowOutputPort=on
  Out1 : Outport
  wires:
  In1/1 -> Out1/1

== system model_min_mine/5 систем підйому/4/7-періодні/7-ми періодна криволінійна/Допоміжний/Генераці ==
  In1 : Inport
  Trigger : TriggerPort  TriggerType=either  VariantControl=(inherit)  ShowOutputPort=on
  Out1 : Outport
  wires:
  In1/1 -> Out1/1

== system model_min_mine/5 систем підйому/4/7-періодні/7-ми періодна криволінійна/Допоміжний1/Генераці ==
  In1 : Inport
  Trigger : TriggerPort  TriggerType=either  VariantControl=(inherit)  ShowOutputPort=on
  Out1 : Outport
  wires:
  In1/1 -> Out1/1

== system model_min_mine/5 систем підйому/4/7-періодні/7-ми періодна пр/Subsystem/Генераці ==
  In1 : Inport
  Trigger : TriggerPort  TriggerType=either  VariantControl=(inherit)  ShowOutputPort=on
  Out1 : Outport
  wires:
  In1/1 -> Out1/1

== system model_min_mine/5 систем підйому/4/7-періодні/7-ми періодна пр/Subsystem1/Генераці ==
  In1 : Inport
  Trigger : TriggerPort  TriggerType=either  VariantControl=(inherit)  ShowOutputPort=on
  Out1 : Outport
  wires:
  In1/1 -> Out1/1

== system model_min_mine/5 систем підйому/4/7-періодні/7-ми періодна пр/Subsystem2/Генераці ==
  In1 : Inport
  Trigger : TriggerPort  TriggerType=either  VariantControl=(inherit)  ShowOutputPort=on
  Out1 : Outport
  wires:
  In1/1 -> Out1/1

== system model_min_mine/5 систем підйому/4/7-періодні/7-ми періодна пр/Subsystem3/Генераці ==
  In1 : Inport
  Trigger : TriggerPort  TriggerType=either  VariantControl=(inherit)  ShowOutputPort=on
  Out1 : Outport
  wires:
  In1/1 -> Out1/1

== system model_min_mine/5 систем підйому/4/7-періодні/7-ми періодна пр/Subsystem6/Генераці ==
  In1 : Inport
  Trigger : TriggerPort  TriggerType=either  VariantControl=(inherit)  ShowOutputPort=on
  Out1 : Outport
  wires:
  In1/1 -> Out1/1

== system model_min_mine/5 систем підйому/4/7-періодні/7-ми періодна пр/Допоміжний/Генераці ==
  In1 : Inport
  Trigger : TriggerPort  TriggerType=either  VariantControl=(inherit)  ShowOutputPort=on
  Out1 : Outport
  wires:
  In1/1 -> Out1/1

== system model_min_mine/5 систем підйому/4/7-періодні/7-ми періодна пр/Допоміжний1/Генераці ==
  In1 : Inport
  Trigger : TriggerPort  TriggerType=either  VariantControl=(inherit)  ShowOutputPort=on
  Out1 : Outport
  wires:
  In1/1 -> Out1/1

== system model_min_mine/5 систем підйому/6/5-періодні/криво/Subsystem/Генераці ==
  In1 : Inport
  Trigger : TriggerPort  TriggerType=either  VariantControl=(inherit)  ShowOutputPort=on
  Out1 : Outport
  wires:
  In1/1 -> Out1/1

== system model_min_mine/5 систем підйому/6/5-періодні/криво/Subsystem1/Генераці ==
  In1 : Inport
  Trigger : TriggerPort  TriggerType=either  VariantControl=(inherit)  ShowOutputPort=on
  Out1 : Outport
  wires:
  In1/1 -> Out1/1

== system model_min_mine/5 систем підйому/6/5-періодні/криво/Subsystem2/Генераці ==
  In1 : Inport
  Trigger : TriggerPort  TriggerType=either  VariantControl=(inherit)  ShowOutputPort=on
  Out1 : Outport
  wires:
  In1/1 -> Out1/1

== system model_min_mine/5 систем підйому/6/5-періодні/криво/Subsystem3/Генераці ==
  In1 : Inport
  Trigger : TriggerPort  TriggerType=either  VariantControl=(inherit)  ShowOutputPort=on
  Out1 : Outport
  wires:
  In1/1 -> Out1/1

== system model_min_mine/5 систем підйому/6/5-періодні/криво/Subsystem6/Генераці ==
  In1 : Inport
  Trigger : TriggerPort  TriggerType=either  VariantControl=(inherit)  ShowOutputPort=on
  Out1 : Outport
  wires:
  In1/1 -> Out1/1

== system model_min_mine/5 систем підйому/6/5-періодні/криво/Допоміжний/Генераці ==
  In1 : Inport
  Trigger : TriggerPort  TriggerType=either  VariantControl=(inherit)  ShowOutputPort=on
  Out1 : Outport
  wires:
  In1/1 -> Out1/1

== system model_min_mine/5 систем підйому/6/5-періодні/криво/Допоміжний1/Генераці ==
  In1 : Inport
  Trigger : TriggerPort  TriggerType=either  VariantControl=(inherit)  ShowOutputPort=on
  Out1 : Outport
  wires:
  In1/1 -> Out1/1

== system model_min_mine/5 систем підйому/6/5-періодні/пр/Subsystem/Генераці ==
  In1 : Inport
  Trigger : TriggerPort  TriggerType=either  VariantControl=(inherit)  ShowOutputPort=on
  Out1 : Outport
  wires:
  In1/1 -> Out1/1

== system model_min_mine/5 систем підйому/6/5-періодні/пр/Subsystem1/Генераці ==
  In1 : Inport
  Trigger : TriggerPort  TriggerType=either  VariantControl=(inherit)  ShowOutputPort=on
  Out1 : Outport
  wires:
  In1/1 -> Out1/1

== system model_min_mine/5 систем підйому/6/5-періодні/пр/Subsystem4/Генераці ==
  In1 : Inport
  Trigger : TriggerPort  TriggerType=either  VariantControl=(inherit)  ShowOutputPort=on
  Out1 : Outport
  wires:
  In1/1 -> Out1/1

== system model_min_mine/5 систем підйому/6/5-періодні/пр/Subsystem5/Генераці ==
  In1 : Inport
  Trigger : TriggerPort  TriggerType=either  VariantControl=(inherit)  ShowOutputPort=on
  Out1 : Outport
  wires:
  In1/1 -> Out1/1

== system model_min_mine/5 систем підйому/6/5-періодні/пр/Subsystem6/Генераці ==
  In1 : Inport
  Trigger : TriggerPort  TriggerType=either  VariantControl=(inherit)  ShowOutputPort=on
  Out1 : Outport
  wires:
  In1/1 -> Out1/1

== system model_min_mine/5 систем підйому/6/5-періодні/пр/Допоміжний/Генераці ==
  In1 : Inport
  Trigger : TriggerPort  TriggerType=either  VariantControl=(inherit)  ShowOutputPort=on
  Out1 : Outport
  wires:
  In1/1 -> Out1/1

== system model_min_mine/5 систем підйому/6/5-періодні/пр/Допоміжний -1/Генераці ==
  In1 : Inport
  Trigger : TriggerPort  TriggerType=either  VariantControl=(inherit)  ShowOutputPort=on
  Out1 : Outport
  wires:
  In1/1 -> Out1/1

== system model_min_mine/5 систем підйому/6/5-періодні/пр/Допоміжний -2/Генераці ==
  In1 : Inport
  Trigger : TriggerPort  TriggerType=either  VariantControl=(inherit)  ShowOutputPort=on
  Out1 : Outport
  wires:
  In1/1 -> Out1/1

== system model_min_mine/5 систем підйому/6/5-періодні/пр/Допоміжний -3/Генераці ==
  In1 : Inport
  Trigger : TriggerPort  TriggerType=either  VariantControl=(inherit)  ShowOutputPort=on
  Out1 : Outport
  wires:
  In1/1 -> Out1/1

== system model_min_mine/5 систем підйому/6/5-періодні/пр/Допоміжний -4/Генераці ==
  In1 : Inport
  Trigger : TriggerPort  TriggerType=either  VariantControl=(inherit)  ShowOutputPort=on
  Out1 : Outport
  wires:
  In1/1 -> Out1/1

== system model_min_mine/5 систем підйому/6/6-періодні/6-ти періодна криволінійна/Subsystem/Генераці ==
  In1 : Inport
  Trigger : TriggerPort  TriggerType=either  VariantControl=(inherit)  ShowOutputPort=on
  Out1 : Outport
  wires:
  In1/1 -> Out1/1

== system model_min_mine/5 систем підйому/6/6-періодні/6-ти періодна криволінійна/Subsystem3/Генераці ==
  In1 : Inport
  Trigger : TriggerPort  TriggerType=either  VariantControl=(inherit)  ShowOutputPort=on
  Out1 : Outport
  wires:
  In1/1 -> Out1/1

== system model_min_mine/5 систем підйому/6/6-періодні/6-ти періодна криволінійна/Subsystem6/Генераці ==
  In1 : Inport
  Trigger : TriggerPort  TriggerType=either  VariantControl=(inherit)  ShowOutputPort=on
  Out1 : Outport
  wires:
  In1/1 -> Out1/1

== system model_min_mine/5 систем підйому/6/6-періодні/6-ти періодна криволінійна/Допоміжний/Генераці ==
  In1 : Inport
  Trigger : TriggerPort  TriggerType=either  VariantControl=(inherit)  ShowOutputPort=on
  Out1 : Outport
  wires:
  In1/1 -> Out1/1

== system model_min_mine/5 систем підйому/6/6-періодні/6-ти періодна криволінійна/Допоміжний1/Генераці ==
  In1 : Inport
  Trigger : TriggerPort  TriggerType=either  VariantControl=(inherit)  ShowOutputPort=on
  Out1 : Outport
  wires:
  In1/1 -> Out1/1

== system model_min_mine/5 систем підйому/6/6-періодні/6-ти періодна пр/Subsystem/Генераці ==
  In1 : Inport
  Trigger : TriggerPort  TriggerType=either  VariantControl=(inherit)  ShowOutputPort=on
  Out1 : Outport
  wires:
  In1/1 -> Out1/1

== system model_min_mine/5 систем підйому/6/6-періодні/6-ти періодна пр/Subsystem1/Генераці ==
  In1 : Inport
  Trigger : TriggerPort  TriggerType=either  VariantControl=(inherit)  ShowOutputPort=on
  Out1 : Outport
  wires:
  In1/1 -> Out1/1

== system model_min_mine/5 систем підйому/6/6-періодні/6-ти періодна пр/Subsystem2/Генераці ==
  In1 : Inport
  Trigger : TriggerPort  TriggerType=either  VariantControl=(inherit)  ShowOutputPort=on
  Out1 : Outport
  wires:
  In1/1 -> Out1/1

== system model_min_mine/5 систем підйому/6/6-періодні/6-ти періодна пр/Subsystem3/Генераці ==
  In1 : Inport
  Trigger : TriggerPort  TriggerType=either  VariantControl=(inherit)  ShowOutputPort=on
  Out1 : Outport
  wires:
  In1/1 -> Out1/1

== system model_min_mine/5 систем підйому/6/6-періодні/6-ти періодна пр/Subsystem6/Генераці ==
  In1 : Inport
  Trigger : TriggerPort  TriggerType=either  VariantControl=(inherit)  ShowOutputPort=on
  Out1 : Outport
  wires:
  In1/1 -> Out1/1

== system model_min_mine/5 систем підйому/6/6-періодні/6-ти періодна пр/Допоміжний/Генераці ==
  In1 : Inport
  Trigger : TriggerPort  TriggerType=either  VariantControl=(inherit)  ShowOutputPort=on
  Out1 : Outport
  wires:
  In1/1 -> Out1/1
